simulink model "Sim_13"  (R2019b)
settings: Solver=VariableStepAuto  StartTime=0.0  StopTime=sim_time  FixedStep=0.01  MaxStep=0.1  MinStep=0.0001  RelTol=0.01  AbsTol=0.01
values from neighbouring files (symbols this model uses):
  Controller_Data = struct('K_p', K_p, 'K_v', K_v, 'K_i', K_i, 'M', M,     'D', D, 'U_ref', U_ref, 'mu', mu)    [Sim_10_init.m]    (also in Sim_11_init.m; Sim_12_init.m; Sim_3_4_and_5_init.m; Sim_7_8_userdef_init.m)
  D = [ 0.66  0    0 ... (first row only)    [Sim_10_init.m]    (also in Sim_11_init.m; Sim_12_init.m; Sim_3_4_and_5_init.m; Sim_7_8_userdef_init.m)
  K_p = 0.08*[1.1  0    0 ... (first row only)    [Sim_10_init.m]    (also in Sim_11_init.m; Sim_12_init.m; Sim_3_4_and_5_init.m; Sim_7_8_userdef_init.m)
  K_v = 1*[10   0       0 ... (first row only)    [Sim_10_init.m]    (also in Sim_11_init.m; Sim_12_init.m; Sim_3_4_and_5_init.m; Sim_7_8_userdef_init.m = 3*[10   0       0)
  LossOfSignalFalse = 1    [Sim_10_init.m]    (also in Sim_11_init.m; Sim_12_init.m; Sim_3_4_and_5_init.m; Sim_7_8_userdef_init.m)
  LossOfSignalTime = 10    [Sim_10_init.m]    (also in Sim_11_init.m; Sim_12_init.m; Sim_3_4_and_5_init.m = 30; Sim_7_8_userdef_init.m)
  LossOfSignalTrue = 0    [Sim_10_init.m]    (also in Sim_11_init.m; Sim_12_init.m; Sim_3_4_and_5_init.m; Sim_7_8_userdef_init.m)
  M = [ 16    0      0 ... (first row only)    [Sim_10_init.m]    (also in Sim_11_init.m; Sim_12_init.m; Sim_3_4_and_5_init.m; Sim_7_8_userdef_init.m)
  mu = 0.09    [Sim_10_init.m]    (also in Sim_11_init.m; Sim_12_init.m; Sim_3_4_and_5_init.m; Sim_7_8_userdef_init.m)
  Observergains = [L1, L2, L3]    [Sim_10_init.m]    (also in Sim_11_init.m; Sim_12_init.m; Sim_3_4_and_5_init.m; Sim_7_8_userdef_init.m)
  path_planner_data = [start_pos; end_pos; Radius; Center]    [Sim_10_init.m]    (also in Sim_11_init.m; Sim_12_init.m; Sim_3_4_and_5_init.m; Sim_7_8_userdef_init.m)
  pathparameter = 0    [Sim_10_init.m]    (also in Sim_11_init.m = 1; Sim_12_init.m; Sim_3_4_and_5_init.m = 1; Sim_7_8_userdef_init.m = 1)
  RegainOfSignalFalse = 0    [Sim_10_init.m]    (also in Sim_11_init.m; Sim_12_init.m; Sim_3_4_and_5_init.m; Sim_7_8_userdef_init.m)
  RegainOfSignalTime = 30    [Sim_10_init.m]    (also in Sim_11_init.m; Sim_12_init.m; Sim_3_4_and_5_init.m = 50; Sim_7_8_userdef_init.m)
  RegainOfSignalTrue = 1    [Sim_10_init.m]    (also in Sim_11_init.m; Sim_12_init.m; Sim_3_4_and_5_init.m; Sim_7_8_userdef_init.m)
  start_pos = [10; 20; pi/2 ]    [Sim_10_init.m]    (also in Sim_11_init.m = [0; 0; 0 ]; Sim_12_init.m = [0; 0; 0 ]; Sim_3_4_and_5_init.m = [0; 0; 0 ]; Sim_7_init.m = [0; 0; 0 ])
undefined symbols (not defined in the file or in its folder): tsamp, WP
(part 3 of 3)

== matlab function Sim_13/Controller/CtrlCustom_SLX/Backstepping controller/S(psi_dot) ==
  data: r input; S_r output
function S_r = fcn(r)
S_r = [ 0  -r   0  ;
         r  0   0   ; 
         0  0   1  ] ;
end

== matlab function Sim_13/Controller/CtrlCustom_SLX/Backstepping controller/Transpose Rotation Matrix ==
  data: psi input; R_psi_trans output
function R_psi_trans = fcn(psi)
R_psi = [ cos(psi)  -sin(psi)   0  ;
                sin(psi)    cos(psi)  0  ; 
                    0              0         1  ] ;
                
R_psi_trans = transpose(R_psi);
end

== matlab function Sim_13/Controller/CtrlCustom_SLX/Backstepping controller/Subsystem/MATLAB Function1 ==
  data: psi input; psi_ref input; psi_ref_new output
function psi_ref_new = ssa( psi, psi_ref)

val1 = psi_ref;
val2 = psi_ref + 2*pi;
val3 = psi_ref - 2*pi;

vals = [val1, val2, val3];

[m, i] = min(abs(vals - psi));

psi_ref_new = vals(i);

== matlab function Sim_13/Controller/CtrlCustom_SLX/Transpose Rotation Matrix ==
  data: psi input; R_psi_trans output
function R_psi_trans = fcn(psi)
R_psi = [ cos(psi)  -sin(psi)   0  ;
                sin(psi)    cos(psi)  0  ; 
                    0              0         1  ] ;
                
R_psi_trans = transpose(R_psi);
end

== matlab function Sim_13/Controller/CtrlCustom_SLX/Backstepping controller/alpha1, z_1 explicit ==
  data: alpha_1 output; eta_d input; eta_df input; eta input; s_dot input; nu_hat input; z_1 output
function [alpha_1, z_1] = fcn(eta_d, eta_df, eta, s_dot, nu_hat)

psi = eta(3);
r = nu_hat(3);

R_psi = [ cos(psi)  -sin(psi)   0  ;
                sin(psi)    cos(psi)  0  ; 
                    0              0         1  ] ;
R_transp = transpose(R_psi);
                
S_r = [ 0  -r   0  ;
         r  0   0   ; 
         0  0   1  ] ;   

[alpha_1, z_1] = -S_r*R_transp*(eta - eta_d) + nu_hat - R_transp*eta_df*s_dot;

== matlab function Sim_13/Controller/CtrlCustom_SLX/Backstepping controller/alpha_1, z_1 - explicit /Rotation Matrix ==
  data: psi input; R_psi output
function R_psi = fcn(psi)
R_psi = [ cos(psi)  -sin(psi)   0  ;
                sin(psi)    cos(psi)  0  ; 
                    0              0         1  ] ;
end

== matlab function Sim_13/Controller/CtrlCustom_SLX/Backstepping controller/d//dt[....] ==
  data: eta input; eta_df input; d_dt output size=3; eta_dff input; nu_hat input; s_dot input; U_s input; U_sf input
function d_dt = fcn(eta, eta_df, eta_dff, nu_hat, s_dot, U_s, U_sf)

psi = eta(3);
r = nu_hat(3);

R_psi = [ cos(psi)  -sin(psi)   0  ;
                sin(psi)    cos(psi)  0  ; 
                    0              0         1  ] ;
R_tr = transpose(R_psi);
                
S_r = [ 0  -r   0  ;
         r  0   0   ; 
         0  0   0  ] ;
     
S_tr = transpose(S_r);

d_dt = S_tr*R_tr*eta_df*U_s + R_tr*s_dot*(eta_dff*U_s + eta_df*U_sf);

== matlab function Sim_13/Controller/CtrlCustom_SLX/Backstepping controller/z_1_dot ==
  data: z_1_dot output size=3; eta_d input; eta_df input; eta input; s_dot input; nu_hat input
function z_1_dot = fcn(eta_d, eta_df, eta, s_dot, nu_hat)

psi = eta(3);
r = nu_hat(3);

R_psi = [ cos(psi)  -sin(psi)   0  ;
                sin(psi)    cos(psi)  0  ; 
                    0              0         1  ] ;
R_transp = transpose(R_psi);
                
S_r = [ 0  -r   0  ;
         r  0   0   ; 
         0  0  0   ] ;   

z_1_dot = -S_r*R_transp*(eta - eta_d) + nu_hat - R_transp*eta_df*s_dot;
